simulink model "Week3_problem3"  (R2020b)
settings: Solver=ode45  StartTime=0.0  StopTime=25  RelTol=1e-3
PreLoadFcn:
  | loadvar
InitFcn:
  | Wheel_Slip=0.2;
  | m=75;
  | R=1.25;
  | g=9.81;
  | I=5;
  | v0=44;
settings Model: Creator=omkar  LastModifiedBy=mluser

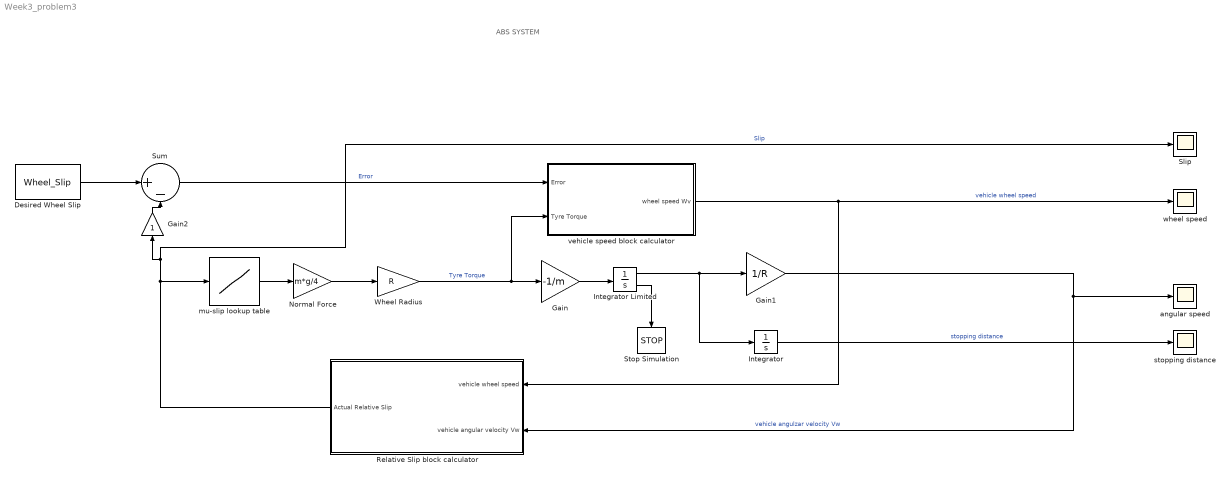
== system Week3_problem3 ==
  note: ABS SYSTEM
  Desired Wheel Slip : Constant  Value=Wheel_Slip
  Gain : Gain  Gain=-1/m
  Gain1 : Gain  Gain=1/R
  Gain2 : Gain
  Integrator : Integrator
  Integrator Limited : Integrator  InitialCondition=v0  LimitOutput=on  UpperSaturationLimit=1000  LowerSaturationLimit=0  ShowSaturationPort=on
  Normal Force : Gain  Gain=m*g/4
  Relative Slip block calculator : Subsystem
  Slip : Scope
  Stop Simulation : Stop
  Sum : Sum  Inputs=|+-
  Wheel Radius : Gain  Gain=R
  angular speed : Scope
  mu-slip lookup table : Lookup_n-D  NumberOfTableDimensions=1  BreakpointsForDimension1=|  Table=|  InternalRulePriority=Speed  RndMeth=Simplest  InputSameDT=on
      BreakpointsForDimension1=|
      | [0
      | 0.05
      | 0.1
      | 0.15
      | 0.2
      | 0.25
      | 0.3
      | 0.35
      | 0.4
      | 0.45
      | 0.5
      | 0.55
      | 0.6
      | 0.65
      | 0.7
      | 0.75
      | 0.8
      | 0.85
      | 0.9
      | 0.95
      | 1
      | ]
      Table=|
      | [0
      | 0.4
      | 0.8
      | 0.97
      | 1
      | 0.98
      | 0.96
      | 0.94
      | 0.92
      | 0.9
      | 0.88
      | 0.855
      | 0.83
      | 0.81
      | 0.79
      | 0.77
      | 0.75
      | 0.73
      | 0.72
      | 0.71
      | 0.7
      | ]
  stopping distance : Scope
  vehicle speed block calculator : Subsystem
      settings: PreSaveFcn=loadvar
  wheel speed : Scope
  wires:
  Desired Wheel Slip/1 -> Sum/1
  Normal Force/1 -> Wheel Radius/1
  mu-slip lookup table/1 -> Normal Force/1
  Sum/1 -> vehicle speed block calculator/1(Error)  "Error"
  Wheel Radius/1 -> Gain/1, vehicle speed block calculator/2(Tyre Torque)  "Tyre Torque"
  vehicle speed block calculator/1(wheel speed Wv) -> Relative Slip block calculator/1(vehicle wheel speed), wheel speed/1  "vehicle wheel speed"
  Gain/1 -> Integrator Limited/1
  Integrator Limited/1 -> Integrator/1, Gain1/1
  Gain1/1 -> Relative Slip block calculator/2(vehicle angular velocity Vw), angular speed/1  "vehicle angulzar velocity Vw"
  Integrator Limited/2 -> Stop Simulation/1
  Integrator/1 -> stopping distance/1  "stopping distance"
  Relative Slip block calculator/1(Actual Relative Slip) -> mu-slip lookup table/1, Gain2/1, Slip/1  "Slip"
  Gain2/1 -> Sum/2

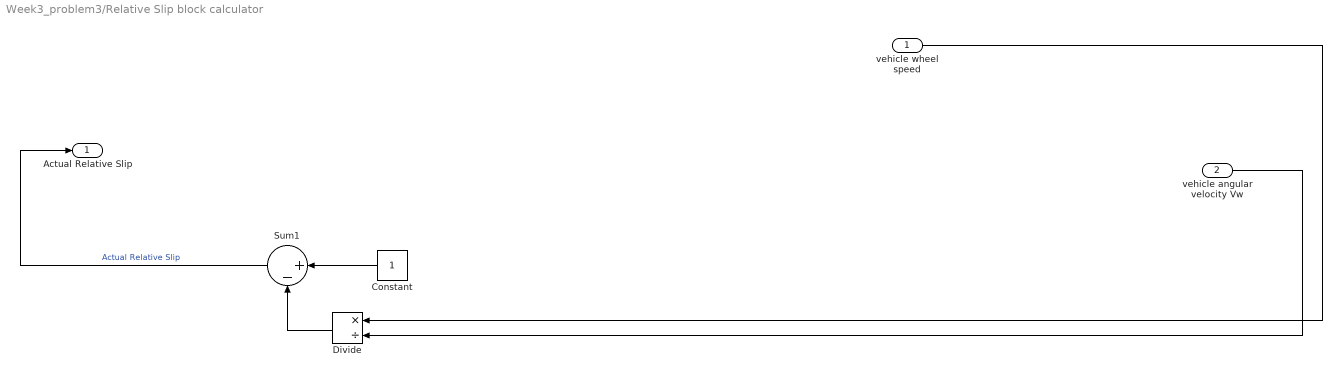
== system Week3_problem3/Relative Slip block calculator ==
  vehicle wheel speed : Inport
  vehicle angular velocity Vw : Inport  Port=2
  Constant : Constant
  Divide : Product  Inputs=*/
  Sum1 : Sum  Inputs=|+-
  Actual Relative Slip : Outport
  wires:
  Constant/1 -> Sum1/1
  Divide/1 -> Sum1/2
  Sum1/1 -> Actual Relative Slip/1  "Actual Relative Slip"
  vehicle angular velocity Vw/1 -> Divide/2
  vehicle wheel speed/1 -> Divide/1

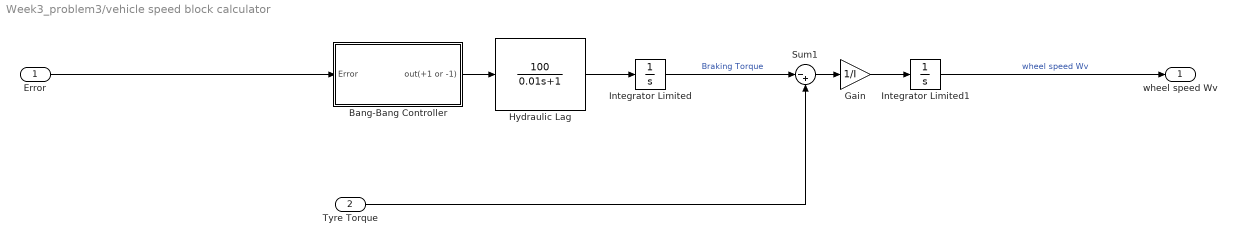
== system Week3_problem3/vehicle speed block calculator ==
  Error : Inport
  Tyre Torque : Inport  Port=2
  Bang-Bang Controller : Subsystem
  Gain : Gain  Gain=1/I
  Hydraulic Lag : TransferFcn  Numerator=[100]  Denominator=[0.01 1]
  Integrator Limited : Integrator  LimitOutput=on  UpperSaturationLimit=1000  LowerSaturationLimit=0
  Integrator Limited1 : Integrator  InitialCondition=v0/R  LimitOutput=on  UpperSaturationLimit=1000  LowerSaturationLimit=0
  Sum1 : Sum  Inputs=|-+
  wheel speed Wv : Outport
  wires:
  Integrator Limited1/1 -> wheel speed Wv/1  "wheel speed Wv"
  Integrator Limited/1 -> Sum1/1  "Braking Torque"
  Gain/1 -> Integrator Limited1/1
  Bang-Bang Controller/1(out(+1 or -1)) -> Hydraulic Lag/1
  Hydraulic Lag/1 -> Integrator Limited/1
  Error/1 -> Bang-Bang Controller/1(Error)
  Tyre Torque/1 -> Sum1/2
  Sum1/1 -> Gain/1

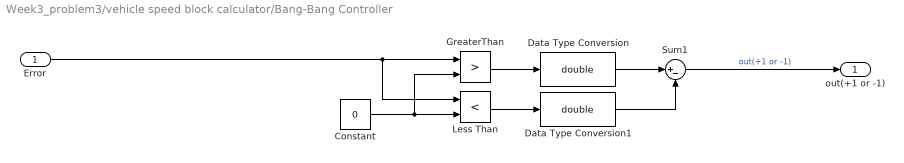
== system Week3_problem3/vehicle speed block calculator/Bang-Bang Controller ==
  Error : Inport
  Constant : Constant  Value=0
  Data Type Conversion : DataTypeConversion  OutDataTypeStr=double  RndMeth=Zero
  Data Type Conversion1 : DataTypeConversion  OutDataTypeStr=double  RndMeth=Zero
  GreaterThan : RelationalOperator  Operator=>  OutDataTypeStr=boolean  RndMeth=Simplest
  Less Than : RelationalOperator  Operator=<  OutDataTypeStr=boolean  RndMeth=Simplest
  Sum1 : Sum  Inputs=|+-
  out(+1 or -1) : Outport
  wires:
  GreaterThan/1 -> Data Type Conversion/1
  Sum1/1 -> out(+1 or -1)/1  "out(+1 or -1)"
  Error/1 -> Less Than/1, GreaterThan/1
  Constant/1 -> GreaterThan/2, Less Than/2
  Data Type Conversion/1 -> Sum1/1
  Data Type Conversion1/1 -> Sum1/2
  Less Than/1 -> Data Type Conversion1/1
